simulink model "sim23"  (R2024a)
settings: Solver=FixedStepAuto  StartTime=0.0  StopTime=70.0  FixedStep=1  RelTol=1e-3
settings Model: Creator=alexe  LastModifiedBy=alexe

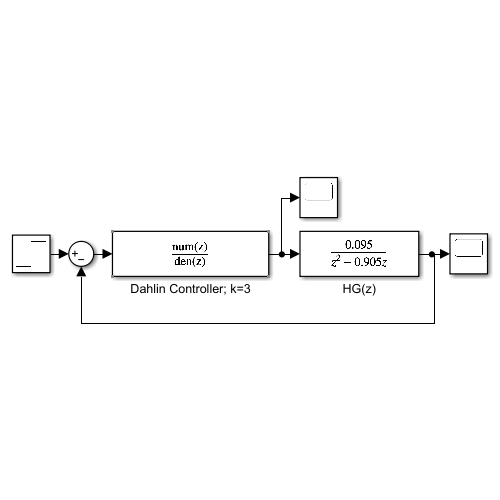
[thumbnail: Simulink's stored preview of the top-level diagram]
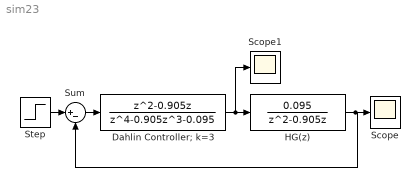
== system sim23 ==
  Dahlin Controller; k=3 : DiscreteTransferFcn  Numerator=[0 0 1 -0.905 0]  Denominator=[1 -0.905 0 0 -0.095]
  HG(z) : DiscreteTransferFcn  Numerator=[0 0 0.095]  Denominator=[1 -0.905 0]
  Scope : Scope
  Scope1 : Scope
  Step : Step
  Sum : Sum  Inputs=|+-
  wires:
  Step/1 -> Sum/1
  Sum/1 -> Dahlin Controller; k=3/1
  Dahlin Controller; k=3/1 -> Scope1/1, HG(z)/1
  HG(z)/1 -> Sum/2, Scope/1
